simulink model "RC_calculation_dongtai_bianjiegou"  (R2023b)
settings: Solver=ode4  StartTime=0.0  StopTime=0.848  FixedStep=0.001  RelTol=1e-3
values from neighbouring files (symbols this model uses):
  a = 4.755148999027856e-06    (= 4.75514899903e-06)    [RC_cal_dongtai_bianjiegou.m]    (also in RC_iden_demo01.m = V(1); RC_iden_demo02.m = V(1))
  a1 = 216.986140271856    (= 216.986140272)    [RC_cal_dongtai_bianjiegou.m]    (also in RC_iden_demo01.m = V(2); RC_iden_demo02.m = V(2))
  a2 = 51.9969921476556    (= 51.9969921477)    [RC_cal_dongtai_bianjiegou.m]    (also in RC_iden_demo01.m = V(3); RC_iden_demo02.m = V(3))
  a3 = -4.667453705814229    (= -4.66745370581)    [RC_cal_dongtai_bianjiegou.m]    (also in RC_iden_demo01.m = V(4); RC_iden_demo02.m = V(4))
  b = -5.745721345365244    (= -5.74572134537)    [RC_cal_dongtai_bianjiegou.m]    (also in RC_iden_Optimization_fmincon_11canshu.m = []; RC_iden_demo01.m = V(5); RC_iden_demo02.m = V(5))
  c1 = 3.69821992974568    (= 3.69821992975)    [RC_cal_dongtai_bianjiegou.m]    (also in RC_iden_demo01.m = V(6); RC_iden_demo02.m = V(6))
  c2 = 8.28628350297708    (= 8.28628350298)    [RC_cal_dongtai_bianjiegou.m]    (also in RC_iden_demo01.m = V(7); RC_iden_demo02.m = V(7))
  c3 = 0.010312630474325    (= 0.0103126304743)    [RC_cal_dongtai_bianjiegou.m]    (also in RC_iden_demo01.m = V(8); RC_iden_demo02.m = V(8))
  f0 = 4.527490174888555    (= 4.52749017489)    [RC_cal_dongtai_bianjiegou.m]    (also in RC_iden_demo01.m = V(9); RC_iden_demo02.m = V(9))
  I = 0.1*i    (= 0)    [RC_cal_dongtai_bianjiegou.m]
  k = -0.017999550541035    (= -0.017999550541)    [RC_cal_dongtai_bianjiegou.m]    (also in RC_iden_demo01.m = V(10); RC_iden_demo02.m = V(10))
  m = 0.019584640303568    (= 0.0195846403036)    [RC_cal_dongtai_bianjiegou.m]    (also in RC_iden_demo01.m = V(11); RC_iden_demo02.m = V(11))
settings Model: Creator=lenovo  LastModifiedBy=Lenovo
settings SolverCC: AlgebraicLoopSolver=TrustRegion  AutoInsertRateTranBlk=on
settings DataIOCC: ReturnWorkspaceOutputs=off
settings OptimizationCC: LifeSpan=inf
settings DebuggingCC: UnconnectedInputMsg=warning  UnconnectedOutputMsg=warning  UnconnectedLineMsg=warning  SFUnexpectedBacktrackingDiag=warning  SFNoUnconditionalDefaultTransitionDiag=warning  SFExecutionAtInitializationDiag=none  ArithmeticOperatorsInVariantConditions=warning
settings ModelReferenceCC: EnableRefExpFcnMdlSchedulingChecks=on
settings SFSimCC: SimUseLocalCustomCode=off  CustomCodeUndefinedFunction=UseInterfaceOnly
settings RTWCC: RTWUseLocalCustomCode=off
settings CodeAppCC: StateflowObjectComments=on
settings GRTTargetCC: TargetLangStandard=C89/C90 (ANSI)
settings ConfigComp: CovMetricSettings=dw  CovSaveCumulativeToWorkspaceVar=on  CovSaveSingleToWorkspaceVar=on  CovExternalEMLEnable=off

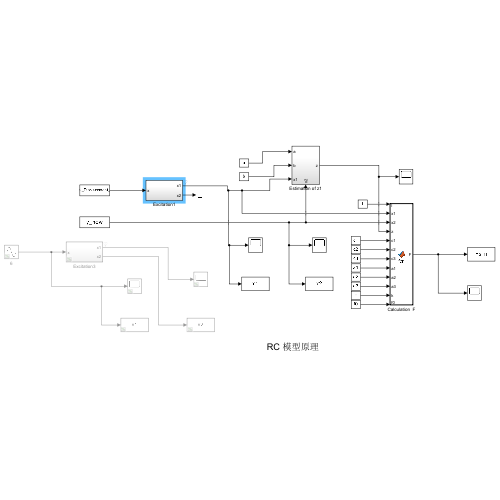
[thumbnail: Simulink's stored preview of the top-level diagram]
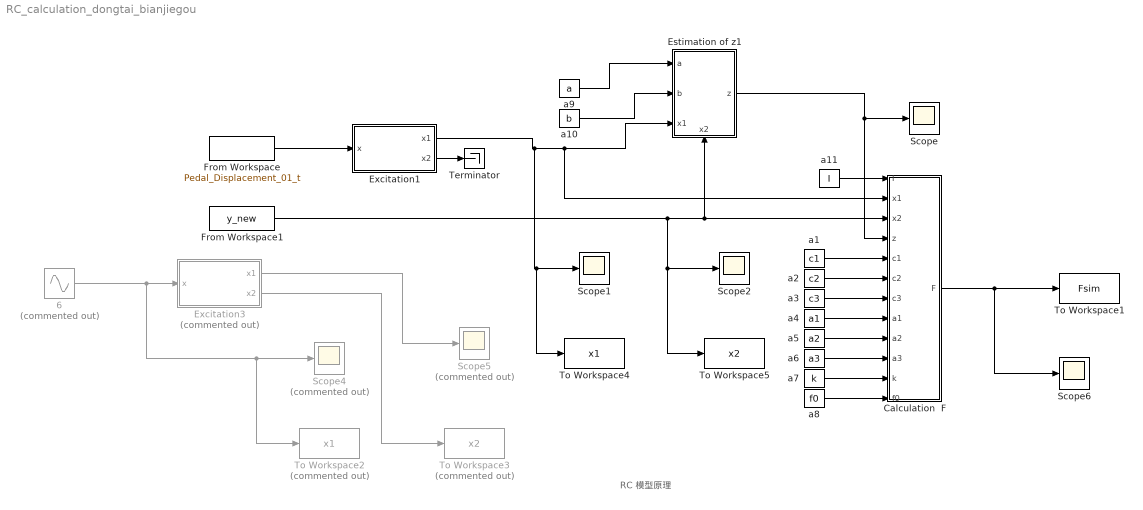
== system RC_calculation_dongtai_bianjiegou ==
  note: RC 模型原理
  6 : Sin  Commented=on  Amplitude=27  Frequency=pi*2  Phase=-pi/2  SampleTime=0
  Calculation  F : MATLAB Function  TreatAsAtomicUnit=on
  Estimation of z1 : Subsystem
      settings: PortSchema="{\"entries\":[{\"content\":{\"sides\":[{\"content\":{\"connectorIds\":[\"In1\",\"In2\",\"In3\"]},\"type\":\"ConnectorPlacement.EquallySpacedRectSide\",\"uuid\":\"2a893864-42cd-4c5d-a3c4-8a16a284f093\"},{\"content\":{\"connectorIds\":[\"Out1\"],\"side\":\"RIGHT\"},\"type\":\"ConnectorPlacement.EquallySpacedRectSide\",\"uuid\":\"28a77d09-70d8-44c2-bc09-b4a5bc86d529\"},{\"content\":{\"side\":\"TOP\"},\"type\":\"ConnectorPlacement.EquallySpacedRectSide\",\"uuid\":\"ab722718-bd7e-4ded-b728-44c927231241\"},{\"content\":{\"connectorIds\":[\"In4\"],\"side\":\"BOTTOM\"},\"type\":\"ConnectorPlacement.EquallySpacedRectSide\",\"uuid\":\"2aab2d18-9074-4c7e-82fb-31ebed71621d\"}]},\"type\":\"ConnectorPlacement.EquallySpacedConnector\",\"uuid\":\"36cf0784-0d02-4874-8e9a-d3ea293461d2\"}],\"packageUris\":[\"http://schema.mathworks.com/mf0/Connector/R2020b\"],\"version\":\"1.0\"}"
  Excitation1 : Subsystem
  Excitation3 : Subsystem  Commented=on
  From Workspace : FromWorkspace  VariableName=Pedal_Displacement_01_t  SampleTime=0.001
  From Workspace1 : FromWorkspace  VariableName=y_new
  Scope{,1..2,6} (4 alike) : Scope
  Scope4 : Scope  Commented=on
  Scope5 : Scope  Commented=on
  Terminator : Terminator
  To Workspace1 : ToWorkspace  VariableName=Fsim  SampleTime=-1
  To Workspace2 : ToWorkspace  Commented=on  VariableName=x1  SampleTime=-1
  To Workspace3 : ToWorkspace  Commented=on  VariableName=x2  SampleTime=-1
  To Workspace4 : ToWorkspace  VariableName=x1  SampleTime=-1
  To Workspace5 : ToWorkspace  VariableName=x2  SampleTime=-1
  a1 : Constant  Value=c1  SampleTime=-1
  a10 : Constant  Value=b  SampleTime=-1
  a11 : Constant  Value=I  SampleTime=-1
  a2 : Constant  Value=c2  SampleTime=-1
  a3 : Constant  Value=c3  SampleTime=-1
  a4 : Constant  Value=a1  SampleTime=-1
  a5 : Constant  Value=a2  SampleTime=-1
  a6 : Constant  Value=a3  SampleTime=-1
  a7 : Constant  Value=k  SampleTime=-1
  a8 : Constant  Value=f0  SampleTime=-1
  a9 : Constant  Value=a  SampleTime=-1
  wires:
  Calculation  F/1(F) -> Scope6/1, To Workspace1/1
  6/1 -> Scope4/1, To Workspace2/1, Excitation3/1(x)
  Excitation3/1(x1) -> Scope5/1
  Estimation of z1/1(z) -> Calculation  F/4(z), Scope/1
  a8/1 -> Calculation  F/12(f0)
  a7/1 -> Calculation  F/11(k)
  a6/1 -> Calculation  F/10(a3)
  a5/1 -> Calculation  F/9(a2)
  a4/1 -> Calculation  F/8(a1)
  a3/1 -> Calculation  F/7(c3)
  a2/1 -> Calculation  F/6(c2)
  a1/1 -> Calculation  F/5(c1)
  a9/1 -> Estimation of z1/1("a ")
  a10/1 -> Estimation of z1/2(b)
  a11/1 -> Calculation  F/1(I)
  Excitation1/1(x1) -> To Workspace4/1, Scope1/1, Calculation  F/2(x1), Estimation of z1/3(x1)
  Excitation3/2(x2) -> To Workspace3/1
  From Workspace/1 -> Excitation1/1(x)
  Excitation1/2(x2) -> Terminator/1
  From Workspace1/1 -> To Workspace5/1, Scope2/1, Estimation of z1/4(x2), Calculation  F/3(x2)

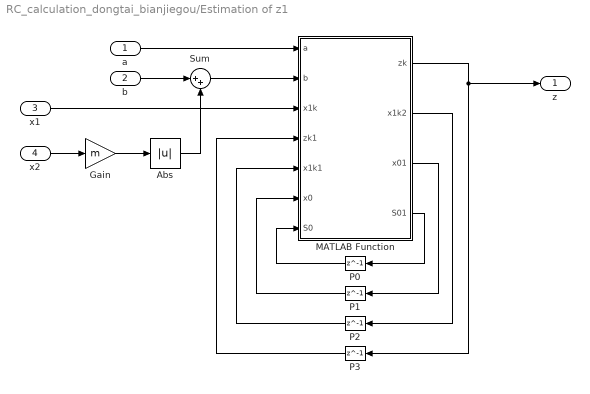
== system RC_calculation_dongtai_bianjiegou/Estimation of z1 ==
  "a " : Inport
  b : Inport  Port=2
  x1 : Inport  Port=3
  x2 : Inport  Port=4
  Abs : Abs  SaturateOnIntegerOverflow=off
  Gain : Gain  Gain=m
  MATLAB Function : MATLAB Function  TreatAsAtomicUnit=on
  P0 : Delay  DelayLength=1  InitialCondition=0.1733
  P1 : Delay  DelayLength=1  InitialCondition=0
  P2 : Delay  DelayLength=1  InitialCondition=0
  P3 : Delay  DelayLength=1  InitialCondition=0
  Sum : Sum  Inputs=|++
  z : Outport
  wires:
  x1/1 -> MATLAB Function/3(x1k)
  MATLAB Function/1(zk) -> z/1, P3/1
  MATLAB Function/4(S01) -> P0/1
  P0/1 -> MATLAB Function/7(S0)
  MATLAB Function/3(x01) -> P1/1
  MATLAB Function/2(x1k2) -> P2/1
  P1/1 -> MATLAB Function/6(x0)
  P2/1 -> MATLAB Function/5(x1k1)
  P3/1 -> MATLAB Function/4(zk1)
  "a "/1 -> MATLAB Function/1(a)
  Gain/1 -> Abs/1
  x2/1 -> Gain/1
  Abs/1 -> Sum/2
  b/1 -> Sum/1
  Sum/1 -> MATLAB Function/2(b)

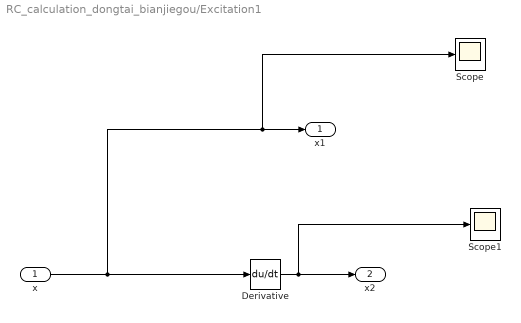
== system RC_calculation_dongtai_bianjiegou/Excitation1 ==
  x : Inport
  Derivative : Derivative
  Scope : Scope
  Scope1 : Scope
  x1 : Outport
  x2 : Outport  Port=2
  wires:
  Derivative/1 -> Scope1/1, x2/1
  x/1 -> Derivative/1, Scope/1, x1/1

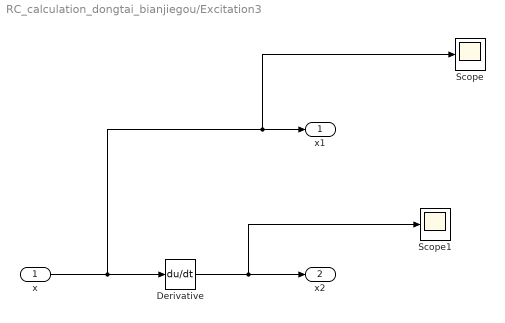
== system RC_calculation_dongtai_bianjiegou/Excitation3 ==
  x : Inport
  Derivative : Derivative
  Scope : Scope
  Scope1 : Scope
  x1 : Outport
  x2 : Outport  Port=2
  wires:
  x/1 -> Derivative/1, Scope/1, x1/1
  Derivative/1 -> Scope1/1, x2/1

== matlab function RC_calculation_dongtai_bianjiegou/Estimation of z1/MATLAB Function ==
  data: a input; b input; zk output; x1k2 output; x1k input; zk1 input; x1k1 input; x0 input; S0 input; x01 output; S01 output
function [zk,x1k2,x01,S01]= fcn(a,b,x1k,zk1,x1k1,x0,S0)


aal=S0*(x1k-x1k1);
    if x1k>x1k1;
        if aal<0;
            S0=(-log((1-zk1)/2)*a)^(1/b);
            x0=x1k1;
            S1=S0+x1k-x0;
        else
            S1=S0+x1k-x0;
        end
        
    elseif x1k<x1k1;
        if aal<0;
            S0=-(abs(log((1+zk1)/2)*a))^(1/b);
            x0=x1k1;
            S1=S0+x1k1-x0;
        else
            S1=S0+x1k1-x0;
        end
    else
        S1=S0+x1k-x0;
    end
       
    if S1>0
        zk=1-2*exp(-S1^b/a);
    else
        zk=-1+2*exp(-(abs(S1))^b/a);
    end
    x1k2=x1k;
    x01=x0;S01=S0;
end

== matlab function RC_calculation_dongtai_bianjiegou/Calculation  F ==
  data: I input; x1 input; x2 input; z input; c1 input; c2 input; c3 input; F output; a1 input; a2 input; a3 input; k input; f0 input
function F = fcn(I,x1,x2,z,c1,c2,c3,a1,a2,a3,k,f0)
%#codegen



F=(c1*I^2+c2*I+c3)*x2+k*x1+(a1*I^2+a2*I+a3)*z+f0;
end
